simulink model "model"  (R2021a)
settings: Solver=VariableStepAuto  StartTime=0.0  StopTime=200  RelTol=1e-3
values from neighbouring files (symbols this model uses):
  A = 2.42    [script.m]
  An = 16    [script.m]
  beta = 0.4    [script.m]
  Cd = 0.32    [script.m]
  Cr = 0.01    [script.m]
  g = 9.80    (= 9.8)    [script.m]
  M = 989    [script.m]
  p = 1.3    [script.m]
  Tmax = 190    [script.m]
  Wmax = 420    [script.m]
undefined symbols (not defined in the file or in its folder): magnitude
settings Model: Creator=marcelo  LastModifiedBy=joao
settings SolverCC: AlgebraicLoopSolver=TrustRegion
settings DebuggingCC: SFMachineParentedDataDiag=warning

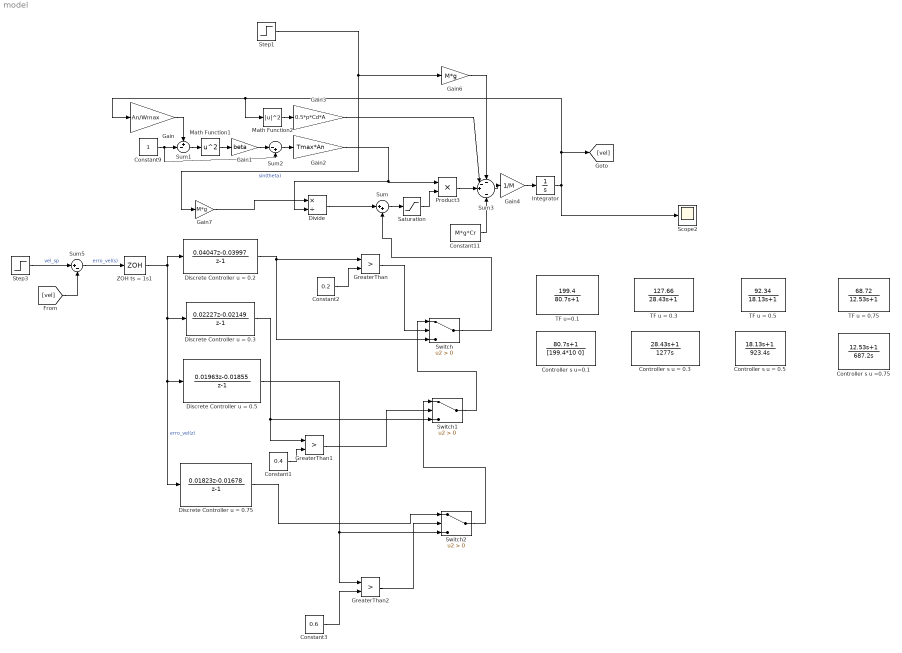
== system model ==
  Constant1 : Constant  Value=0.4
  Constant11 : Constant  Value=M*g*Cr
  Constant2 : Constant  Value=0.2
  Constant3 : Constant  Value=0.6
  Constant9 : Constant
  Controller s u = 0.3 : TransferFcn  Numerator=[28.43 1]  Denominator=[1277 0]
  Controller s u = 0.5 : TransferFcn  Numerator=[18.13 1]  Denominator=[923.4 0]
  Controller s u =0.75 : TransferFcn  Numerator=[12.53 1]  Denominator=[687.2 0]
  Controller s u=0.1 : TransferFcn  Numerator=[80.7 1]  Denominator=[199.4*10 0]
  Discrete Controller u = 0.2 : DiscreteTransferFcn  Numerator=[0.04047 -0.03997]  Denominator=[1 -1]
  Discrete Controller u = 0.3 : DiscreteTransferFcn  Numerator=[0.02227 -0.02149]  Denominator=[1 -1]
  Discrete Controller u = 0.5 : DiscreteTransferFcn  Numerator=[0.01963 -0.01855]  Denominator=[1 -1]
  Discrete Controller u = 0.75 : DiscreteTransferFcn  Numerator=[0.01823 -0.01678]  Denominator=[1 -1]
  Divide : Product  Inputs=*/
  Gain : Gain  Gain=An/Wmax
  Gain1 : Gain  Gain=beta
  Gain2 : Gain  Gain=Tmax*An
  Gain3 : Gain  Gain=0.5*p*Cd*A
  Gain4 : Gain  Gain=1/M
  Gain6 : Gain  Gain=M*g
  Gain7 : Gain  Gain=M*g
  GreaterThan : RelationalOperator  Operator=>  OutDataTypeStr=boolean  RndMeth=Simplest
  GreaterThan1 : RelationalOperator  Operator=>  OutDataTypeStr=boolean  RndMeth=Simplest
  GreaterThan2 : RelationalOperator  Operator=>  OutDataTypeStr=boolean  RndMeth=Simplest
  Integrator : Integrator
  Math Function1 : Math  Operator=square  SaturateOnIntegerOverflow=on
  Math Function2 : Math  Operator=magnitude^2  SaturateOnIntegerOverflow=on
  Product3 : Product
  Saturation : Saturate  UpperLimit=1  LowerLimit=0
  Scope2 : Scope
  Step1 : Step  Time=5  After=0.2  SampleTime=0
  Step3 : Step  After=20  SampleTime=0
  Sum : Sum  Inputs=|++
  Sum1 : Sum  Inputs=+-|
  Sum2 : Sum  Inputs=|-+
  Sum3 : Sum  Inputs=--+|-
  Sum5 : Sum  Inputs=|+-
  Switch : Switch  Criteria=u2 > Threshold
  Switch1 : Switch  Criteria=u2 > Threshold
  Switch2 : Switch  Criteria=u2 > Threshold
  TF u = 0.3 : TransferFcn  Numerator=[127.66]  Denominator=[28.43 1]
  TF u = 0.5 : TransferFcn  Numerator=[92.34]  Denominator=[18.13 1]
  TF u = 0.75 : TransferFcn  Numerator=[68.72]  Denominator=[12.53 1]
  TF u=0.1 : TransferFcn  Numerator=[199.4]  Denominator=[80.7 1]
  ZOH ts = 1s1 : ZeroOrderHold
  wires:
  Gain4/1 -> Integrator/1
  Constant9/1 -> Sum2/2, Sum1/2
  Gain/1 -> Sum1/1
  Sum1/1 -> Math Function1/1
  Math Function1/1 -> Gain1/1
  Gain1/1 -> Sum2/1
  Sum2/1 -> Gain2/1
  Discrete Controller u = 0.2/1 -> Switch/3, GreaterThan/1
  Math Function2/1 -> Gain3/1
  Gain3/1 -> Sum3/2
  Product3/1 -> Sum3/3
  Constant11/1 -> Sum3/4
  Sum3/1 -> Gain4/1
  Step1/1 -> Gain6/1, Gain7/1  "sin(theta)"
  Gain6/1 -> Sum3/1
  Saturation/1 -> Product3/2
  Constant2/1 -> GreaterThan/2
  GreaterThan/1 -> Switch/2
  Switch/1 -> Sum/2
  ZOH ts = 1s1/1 -> Discrete Controller u = 0.75/1, Discrete Controller u = 0.5/1, Discrete Controller u = 0.3/1, Discrete Controller u = 0.2/1  "erro_vel(z)"
  Step3/1 -> Sum5/1  "vel_sp"
  Sum5/1 -> ZOH ts = 1s1/1  "erro_vel(s)"
  Integrator/1 -> Scope2/1, [vel], Math Function2/1, Gain/1
  [vel] -> Sum5/2
  Discrete Controller u = 0.3/1 -> GreaterThan1/1, Switch1/3
  GreaterThan1/1 -> Switch1/2
  Constant1/1 -> GreaterThan1/2
  Discrete Controller u = 0.5/1 -> GreaterThan2/1, Switch2/3
  Switch1/1 -> Switch/1
  GreaterThan2/1 -> Switch2/2
  Constant3/1 -> GreaterThan2/2
  Discrete Controller u = 0.75/1 -> Switch2/1
  Switch2/1 -> Switch1/1
  Gain2/1 -> Divide/2, Product3/1
  Sum/1 -> Saturation/1
  Gain7/1 -> Divide/1
  Divide/1 -> Sum/1
